simulink subsystem "SubSystemHubmagnet"  (R2020b)
settings: Solver=VariableStepAuto  StartTime=0.0  StopTime=10.0  RelTol=1e-3
settings Model: Creator=kaebi  LastModifiedBy=kaebi

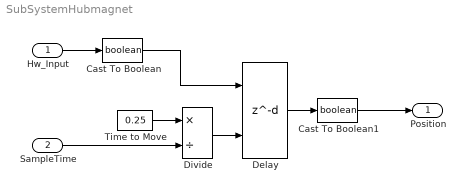
== system SubSystemHubmagnet ==
  Hw_Input : Inport
  SampleTime : Inport  Port=2
  Cast To Boolean : DataTypeConversion  OutDataTypeStr=boolean
  Cast To Boolean1 : DataTypeConversion  OutDataTypeStr=boolean
  Delay : Delay  DelayLengthSource=Input port  DelayLengthUpperLimit=2500
      settings: InputPortMap=u0,p1
  Divide : Product  Inputs=*/
  Time to Move : Constant  Value=0.25
  Position : Outport
  wires:
  SampleTime/1 -> Divide/2
  Time to Move/1 -> Divide/1
  Divide/1 -> Delay/2
  Delay/1 -> Cast To Boolean1/1
  Hw_Input/1 -> Cast To Boolean/1
  Cast To Boolean/1 -> Delay/1
  Cast To Boolean1/1 -> Position/1
